simulink model "model5points"  (R2020b)
settings: Solver=VariableStepAuto  StartTime=0.0  StopTime=10  RelTol=1e-3
model workspace (MAT data in the model file):
  B = 0.169
  Kf = 0.001
  r = 0.027
values from neighbouring files (symbols this model uses):
  J = 0.002437632    [graphics.m]
  ke = 0.48756937411725393    (= 0.487569374117)    [graphics.m]
  km = ke    (= 0.487569374117)    [graphics.m]
  L = 0.0047    [graphics.m]
  R = 8.183683911882799    (= 8.18368391188)    [graphics.m]
undefined symbols (not defined in the file or in its folder): magnitude
settings Model: Creator=spide  LastModifiedBy=vital

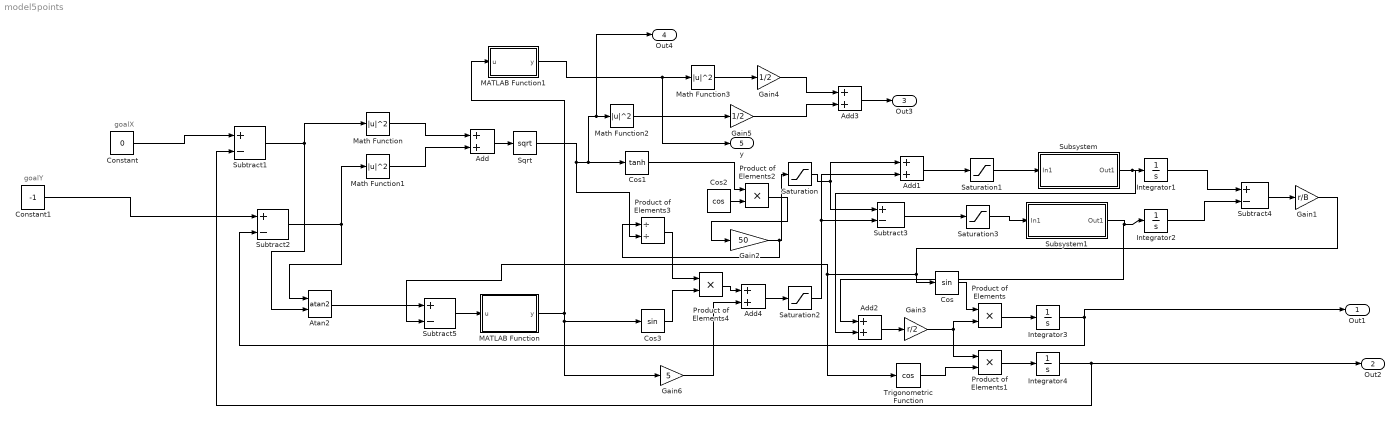
== system model5points ==
  note: goalY
  note: goalX
  Add{,1..4} (5 alike) : Sum
  Atan2 : Trigonometry  Operator=atan2
  Constant : Constant  Value=0
  Constant1 : Constant  Value=-1
  Cos : Trigonometry
  Cos1 : Trigonometry  Operator=tanh
  Cos2 : Trigonometry  Operator=cos
  Cos3 : Trigonometry
  Gain1 : Gain  Gain=r/B
  Gain2 : Gain  Gain=50
  Gain3 : Gain  Gain=r/2
  Gain4 : Gain  Gain=1/2
  Gain5 : Gain  Gain=1/2
  Gain6 : Gain  Gain=5
  Integrator{1..4} (4 alike) : Integrator
  MATLAB Function : MATLAB Function  TreatAsAtomicUnit=on
  MATLAB Function1 : MATLAB Function  TreatAsAtomicUnit=on
  Math Function{,1..3} (4 alike) : Math  Operator=magnitude^2  SaturateOnIntegerOverflow=on
  Product of Elements{,1..2,4} (4 alike) : Product  Inputs=**
  Product of Elements3 : Product  Inputs=//
  Saturation : Saturate  UpperLimit=6  LowerLimit=-6
  Saturation1 : Saturate  UpperLimit=8  LowerLimit=-8
  Saturation2 : Saturate  UpperLimit=2  LowerLimit=-2
  Saturation3 : Saturate  UpperLimit=8  LowerLimit=-8
  Sqrt : Sqrt  SaturateOnIntegerOverflow=on
  Subsystem : Subsystem
  Subsystem1 : Subsystem
  Subtract{1..5} (5 alike) : Sum  Inputs=+-
  Trigonometric Function : Trigonometry  Operator=cos
  Out1 : Outport  SignalName=Y
  Out2 : Outport  Port=2  SignalName=X
  Out3 : Outport  Port=3  SignalName=V
  Out4 : Outport  Port=4  SignalName=p
  y : Outport  Port=5  SignalName=a
  wires:
  Math Function/1 -> Add/1
  Math Function1/1 -> Add/2
  Add/1 -> Sqrt/1
  Sqrt/1 -> Product of Elements3/2, Cos1/1, Out4/1, Math Function2/1
  Saturation/1 -> Subtract3/1, Add1/1
  Add1/1 -> Saturation1/1
  Subtract3/1 -> Saturation3/1
  Saturation1/1 -> Subsystem/1(In1)
  Saturation3/1 -> Subsystem1/1(In1)
  Subsystem/1(Out1) -> Add2/2, Integrator1/1
  Integrator1/1 -> Subtract4/1
  Subsystem1/1(Out1) -> Add2/1, Integrator2/1
  Integrator2/1 -> Subtract4/2
  Subtract4/1 -> Gain1/1
  Atan2/1 -> Subtract5/1
  MATLAB Function/1(y) -> MATLAB Function1/1(u), Gain6/1, Cos3/1
  Saturation2/1 -> Subtract3/2, Add1/2
  Add2/1 -> Gain3/1
  Cos/1 -> Product of Elements/1
  Gain3/1 -> Product of Elements1/1, Product of Elements/2
  Trigonometric Function/1 -> Product of Elements1/2
  Product of Elements/1 -> Integrator3/1
  Product of Elements1/1 -> Integrator4/1
  Gain1/1 -> Subtract5/2, Trigonometric Function/1, Cos/1
  Subtract2/1 -> Atan2/1, Math Function1/1
  Subtract1/1 -> Math Function/1, Atan2/2
  Subtract5/1 -> MATLAB Function/1(u)
  Constant/1 -> Subtract1/1
  Constant1/1 -> Subtract2/1
  Integrator4/1 -> Out2/1, Subtract1/2
  Integrator3/1 -> Out1/1, Subtract2/2
  Math Function3/1 -> Gain4/1
  Math Function2/1 -> Gain5/1
  Gain4/1 -> Add3/1
  Gain5/1 -> Add3/2
  Add3/1 -> Out3/1
  Cos1/1 -> Product of Elements2/1
  Cos2/1 -> Product of Elements2/2
  Product of Elements2/1 -> Gain2/1
  Gain2/1 -> Product of Elements3/1, Saturation/1
  Product of Elements3/1 -> Product of Elements4/1
  Cos3/1 -> Product of Elements4/2
  Product of Elements4/1 -> Add4/1
  Gain6/1 -> Add4/2
  Add4/1 -> Saturation2/1
  MATLAB Function1/1(y) -> y/1, Math Function3/1

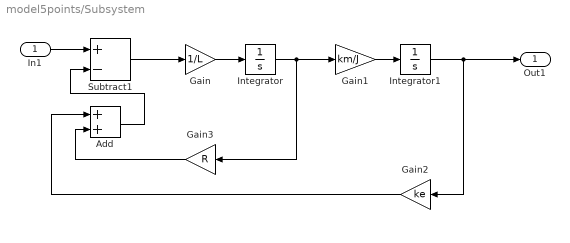
== system model5points/Subsystem ==
  In1 : Inport
  Add : Sum
  Gain : Gain  Gain=1/L
  Gain1 : Gain  Gain=km/J
  Gain2 : Gain  Gain=ke
  Gain3 : Gain  Gain=R
  Integrator : Integrator
  Integrator1 : Integrator
  Subtract1 : Sum  Inputs=+-
  Out1 : Outport
  wires:
  In1/1 -> Subtract1/1
  Add/1 -> Subtract1/2
  Subtract1/1 -> Gain/1
  Gain/1 -> Integrator/1
  Gain3/1 -> Add/2
  Integrator/1 -> Gain3/1, Gain1/1
  Gain1/1 -> Integrator1/1
  Integrator1/1 -> Out1/1, Gain2/1
  Gain2/1 -> Add/1

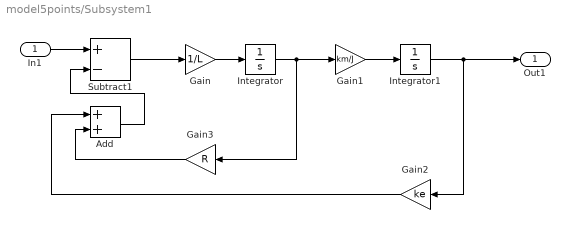
== system model5points/Subsystem1 ==
  In1 : Inport
  Add : Sum
  Gain : Gain  Gain=1/L
  Gain1 : Gain  Gain=km/J
  Gain2 : Gain  Gain=ke
  Gain3 : Gain  Gain=R
  Integrator : Integrator
  Integrator1 : Integrator
  Subtract1 : Sum  Inputs=+-
  Out1 : Outport
  wires:
  In1/1 -> Subtract1/1
  Add/1 -> Subtract1/2
  Subtract1/1 -> Gain/1
  Gain/1 -> Integrator/1
  Gain3/1 -> Add/2
  Integrator/1 -> Gain3/1, Gain1/1
  Gain1/1 -> Integrator1/1
  Integrator1/1 -> Out1/1, Gain2/1
  Gain2/1 -> Add/1

== matlab function model5points/MATLAB Function ==
  data: u input; y output
function y = fcn(u)
if (u > 0)
    if (abs(u) > pi)
    if (abs(u) < 2*pi)
        u = -2*pi + u;
    end
    end
elseif (u < 0)
    if (abs(u) > pi)
        if (abs(u) < 2*pi)
            u = 2*pi + u;
        end
    end
end
y = u;

== matlab function model5points/MATLAB Function1 ==
  data: u input; y output
function y = fcn(u)
if (abs(abs(u) - 2*pi)< 0.0000001)
    u = 0;
end
y = u;
